simulink model "m702"  (Simulink 6.1)
settings: Solver=ode45  StartTime=0.0  StopTime=10.0  RelTol=1e-3
settings Model: LastModifiedBy=okawa
settings DebuggingCC: SolverPrmCheckMsg=warning

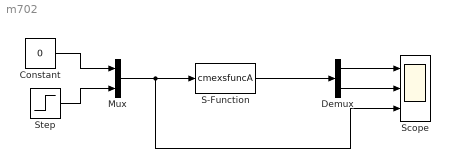
== system m702 ==
  Constant : Constant  Value=0
  Demux : Demux  Outputs=2
  Mux : Mux  Inputs=2
  S-Function : S-Function  FunctionName=cmexsfuncA
  Scope : Scope  NumInputPorts=3
      settings: YMin=-5~-5~-5  YMax=5~5~5
  Step : Step  SampleTime=0
  wires:
  Constant/1 -> Mux/1
  Step/1 -> Mux/2
  Mux/1 -> S-Function/1, Scope/3
  S-Function/1 -> Demux/1
  Demux/1 -> Scope/1
  Demux/2 -> Scope/2
